simulink model "AUV_NDI"  (R2019b)
settings: Solver=VariableStepAuto  StartTime=0.0  StopTime=10.0  RelTol=1e-3
settings Model: Creator=7385281  LastModifiedBy=7385281

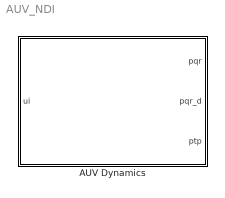
== system AUV_NDI ==
  AUV Dynamics : Subsystem

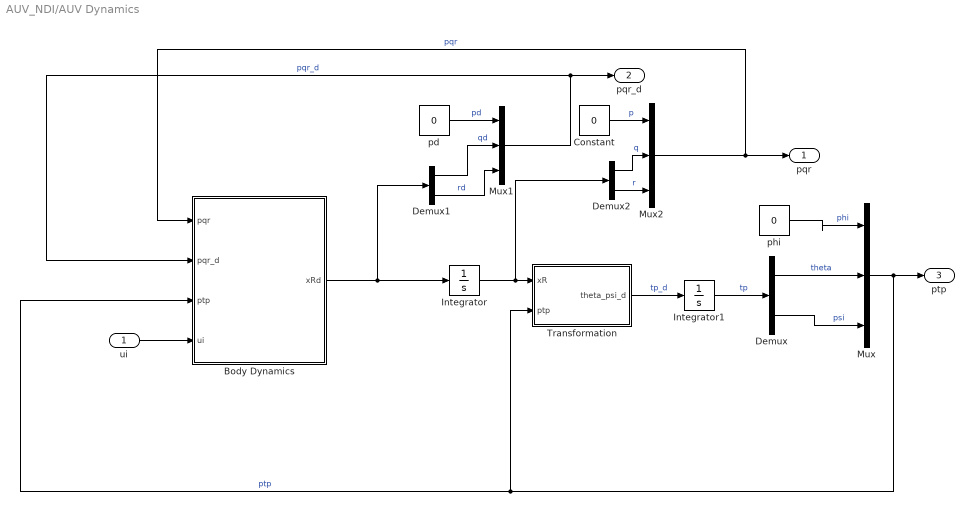
== system AUV_NDI/AUV Dynamics ==
  ui : Inport
  Body Dynamics : MATLAB Function  TreatAsAtomicUnit=on
  Constant : Constant  Value=0
  Demux : Demux  Outputs=2
  Demux1 : Demux  Outputs=2
  Demux2 : Demux  Outputs=2
  Integrator : Integrator  InitialCondition=[0.0001; 0.0001]
  Integrator1 : Integrator
  Mux : Mux  Inputs=3
  Mux1 : Mux  Inputs=3
  Mux2 : Mux  Inputs=3
  Transformation : MATLAB Function  TreatAsAtomicUnit=on
  pd : Constant  Value=0
  phi : Constant  Value=0
  pqr : Outport
  pqr_d : Outport  Port=2
  ptp : Outport  Port=3
  wires:
  Integrator1/1 -> Demux/1  "tp"
  Mux1/1 -> pqr_d/1, Body Dynamics/2(pqr_d)  "pqr_d"
  Demux/1 -> Mux/2  "theta"
  Integrator/1 -> Demux2/1, Transformation/1(xR)
  Mux/1 -> Body Dynamics/3(ptp), Transformation/2(ptp), ptp/1  "ptp"
  Demux2/2 -> Mux2/3  "r"
  Body Dynamics/1(xRd) -> Demux1/1, Integrator/1
  ui/1 -> Body Dynamics/4(ui)
  Demux1/2 -> Mux1/3  "rd"
  pd/1 -> Mux1/1  "pd"
  Demux/2 -> Mux/3  "psi"
  Demux1/1 -> Mux1/2  "qd"
  phi/1 -> Mux/1  "phi"
  Demux2/1 -> Mux2/2  "q"
  Transformation/1(theta_psi_d) -> Integrator1/1  "tp_d"
  Mux2/1 -> pqr/1, Body Dynamics/1(pqr)  "pqr"
  Constant/1 -> Mux2/1  "p"

== matlab function AUV_NDI/AUV Dynamics/Transformation ==
  data: xR input; theta_psi_d output; ptp input
function theta_psi_d = fcn(xR,ptp)
%{
INOFRMATION
    Title: Angle Transformation
    Author: Ben Colvin
    Project: AUV_NDI
    % Date: 12/14/2020

DESCRIPTION:
    This function converts the body rate dynamics to the world-frame
    orientation angles derivative

INPUTS:
    xR - 2x1 vector of body rate dynamics [q r]'
    ptp - 3x1 vector of world orientation angles

OUTPUTS:
    theta_psi_d - 2x1 vector of the derivatives of the world frame 
        angles vector [q r]' 
%}

% CONSTANTS:

% Body Rate Dynamics
q = xR(1);
r = xR(2);

% World Orientation
phi = ptp(1);
theta = ptp(2);
psi = ptp(3);

% Transformation Matrix
H = [cos(phi) -sin(phi); sin(phi)/cos(theta) cos(phi)/cos(phi)];

% Convert body rate dynamics to body Euler angle rates theta and psi
theta_psi_d = H*[q; r];

== matlab function AUV_NDI/AUV Dynamics/Body Dynamics ==
  data: pqr input; xRd output; pqr_d input; ptp input; ui input
function xRd = fcn(pqr,pqr_d,ptp,ui)
%{
INOFRMATION
    Title: Body Rate Dynamics
    Author: Ben Colvin
    Project: AUV_NDI
    % Date: 12/14/2020

DESCRIPTION:
    This function simulates the dynamics of the AUV and how it moves in
    its enviroment.

INPUTS:
    pqr - 3x1 vector of body rotation speeds
    pqr_d - 3x1 vector, derivative of pqr
    ptp - 3x1 vector of world orientation angles
    ui - 2x1 control vector

OUTPUTS:
    xRd - 2x1 vector of the derivatives of the body rate 
        state vector [q r]' 
%}
% CONSTANTS:

% INPUT PARAMETERS
% Sets variables from vectors
p = pqr(1);
q = pqr(2);
r = pqr(3);

pd = pqr_d(1);
qd = pqr_d(2);
rd = pqr_d(3);

phi = ptp(1);
theta = ptp(2);
psi = ptp(3);

% Body Rates State Vector
xR = [q; r];

A1 = -(((Ix-Iz)*r*p+m*(zg*(ud-v*r+w*q)-xg*(wd-u*q+v*p)))+Mqd*qd+Mwd*wd+...
    Mrp*r*p+Mq*u*q)/(Iy-Mqd)+(Mw*u*w+Mww*w*abs(w)+Mqq*q*abs(q)-(xg*W-xb*B)...
    *cos(theta)*cos(phi)-(zg*W-zb*B)*sin(theta))/(Iy-Mqd);

A2 = -(((Iy-Ix)*p*q+m*(xg*(vd-w*p+u*r)-yg*(ud-v*r+w*q)))+Nrd*rd+Nvd*vd+...
    Npq*p*q+Nr*u*r)/(Iz-Nrd)+(Nv*u*v+Nrr*r*abs(r)+Nvv*v&abs(v)-(xg*W-xb*B)...
    *cos(theta)*sin(phi)+(yg*W-yb*B)*sin(theta))/(Iz-Nrd);
    
Ar = [A1; A2];

Br = [0 -Tp*xR/(Iy-Mqd) 0; 0 0 Tp*xR/(Iz-Nrd)];


% The Differential Equation of the body rate dynamics xRd is: xRd =
% Ar+Br*ui
xRd = Ar+Br*ui;
